simulink model "Project_Simulation"  (R2020a)
settings: Solver=ode45  StartTime=0.0  StopTime=1  RelTol=1e-3
libraries: powerlib x17, re_lib x1, simulink x1
settings Model: Creator=Kryptic  LastModifiedBy=Kryptic

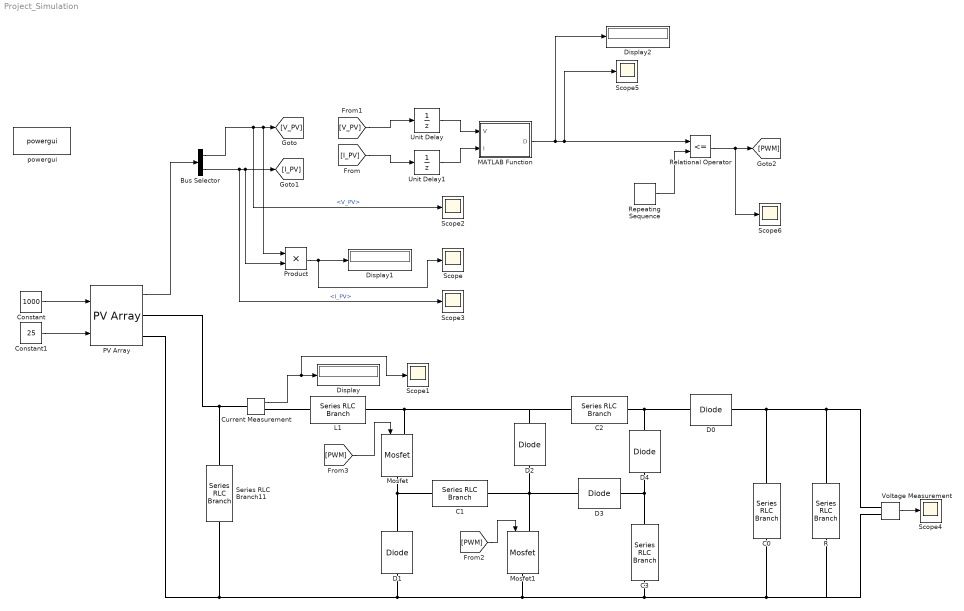
== system Project_Simulation ==
  Bus Selector : BusSelector  OutputSignals=V_PV,I_PV
  C0 : powerlib/Elements/Series RLC Branch  LConnTagsString=__new0  RConnTagsString=__new0  BranchType=C  Resistance=1  Inductance=1e-3  SetiL0=off  InitialCurrent=0  Capacitance=9.82e-8  Setx0=off  InitialVoltage=0  Measurements=None
  C1 : powerlib/Elements/Series RLC Branch  LConnTagsString=__new0  RConnTagsString=__new0  BranchType=C  Resistance=1  Inductance=1e-3  SetiL0=off  InitialCurrent=0  Capacitance=4.74e-6  Setx0=off  InitialVoltage=0  Measurements=None
  C2 : powerlib/Elements/Series RLC Branch  LConnTagsString=__new0  RConnTagsString=__new0  BranchType=C  Resistance=1  Inductance=1e-3  SetiL0=off  InitialCurrent=0  Capacitance=3.75e-7  Setx0=off  InitialVoltage=0  Measurements=None
  C3 : powerlib/Elements/Series RLC Branch  LConnTagsString=__new0  RConnTagsString=__new0  BranchType=C  Resistance=1  Inductance=1e-3  SetiL0=off  InitialCurrent=0  Capacitance=7.5e-7  Setx0=off  InitialVoltage=0  Measurements=None
  Constant : Constant  Value=1000
  Constant1 : Constant  Value=25
  Current Measurement : powerlib/Measurements/Current Measurement  PhasorSimulation=off  OutputType=Complex  PSBequivalent=0
  D0 : powerlib/Power Electronics/Diode  Ron=0.001  Lon=0  Vf=1.50  IC=0  UseSnubber=0  Rs=500  Cs=250e-9  Measurements=off
  D1 : powerlib/Power Electronics/Diode  Ron=0.001  Lon=0  Vf=0.86  IC=0  UseSnubber=0  Rs=500  Cs=250e-9  Measurements=off
  D2 : powerlib/Power Electronics/Diode  Ron=0.001  Lon=0  Vf=0.86  IC=0  UseSnubber=0  Rs=500  Cs=250e-9  Measurements=off
  D3 : powerlib/Power Electronics/Diode  Ron=0.001  Lon=0  Vf=0.86  IC=0  UseSnubber=0  Rs=500  Cs=250e-9  Measurements=off
  D4 : powerlib/Power Electronics/Diode  Ron=0.001  Lon=0  Vf=1.50  IC=0  UseSnubber=0  Rs=500  Cs=250e-9  Measurements=off
  Display : Display
  Display1 : Display
  Display2 : Display
  L1 : powerlib/Elements/Series RLC Branch  LConnTagsString=__new0  RConnTagsString=__new0  BranchType=L  Resistance=1  Inductance=20e-3  SetiL0=off  InitialCurrent=0  Capacitance=1e-6  Setx0=off  InitialVoltage=0  Measurements=None
  MATLAB Function : MATLAB Function  TreatAsAtomicUnit=on
  Mosfet : powerlib/Power Electronics/Mosfet  Ron=8e-3  Lon=0  Rd=0.01  Vfd=0  IC=0  Rs=1e5  Cs=inf  Measurements=off
  Mosfet1 : powerlib/Power Electronics/Mosfet  Ron=8e-3  Lon=0  Rd=0.01  Vfd=0  IC=0  Rs=1e5  Cs=inf  Measurements=off
  PV Array : re_lib/Solar/PV Array  Npar=1  Nser=1  PlotType=array @ 25 deg.C & specified irradiances  S_vec="[ 1000  500  100 ]"  Temp_C_vec="[ 45 25  ]"  ModuleName=User-defined  PlotWhenSelected=off  Pm=20.06  Ncell=60  Voc=21  Isc=1.2  Vm=17  Im=1.18  beta_Voc_pc=-.585  alpha_Isc_pc=0.00367  beta_Voc=-0.12285  alpha_Isc=4.404e-05  IL=1.2439  I0=1.4121e-08  nI=0.7447  Rsh=22939.389  Rs=0.77008  RobustModel=off  RobustCellTemperature=25  BAL=on  Tc=1e-6  Tfilter=5e-5
  Product : Product
  R : powerlib/Elements/Series RLC Branch  LConnTagsString=__new0  RConnTagsString=__new0  BranchType=R  Resistance=2645  Inductance=1e-3  SetiL0=off  InitialCurrent=0  Capacitance=1e-6  Setx0=off  InitialVoltage=0  Measurements=None
  Relational Operator : RelationalOperator  Operator=<=  OutDataTypeStr=boolean  RndMeth=Simplest
  Repeating Sequence : simulink/Sources/Repeating Sequence  rep_seq_t=[0 1/30000]  rep_seq_y=[0 1]
  Scope{,1..6} (7 alike) : Scope
  Series RLC Branch11 : powerlib/Elements/Series RLC Branch  LConnTagsString=__new0  RConnTagsString=__new0  BranchType=RC  Resistance=0.0001  Inductance=1e-3  SetiL0=off  InitialCurrent=0  Capacitance=1000e-6  Setx0=off  InitialVoltage=0  Measurements=None
  Unit Delay : UnitDelay  SampleTime=1e-4  HasFrameUpgradeWarning=on
  Unit Delay1 : UnitDelay  SampleTime=1e-4  HasFrameUpgradeWarning=on
  Voltage Measurement : powerlib/Measurements/Voltage Measurement  PhasorSimulation=off  OutputType=Complex  PSBequivalent=0
  powergui : powerlib/powergui  Priority=1  SimulationMode=Discrete  SampleTime=1e-6  frequency=60  Iterations=50  frequencyindice=0  Pbase=100e6  ErrMax=1e-4  UnitsV=kV  UnitsW=MW  buscounter=0  FunctionMessages=off  echomessages=off  EnableUseOfTLC=off  CurrentSourceSwitches=off  DisableSnubberDevices=off  DisableRonSwitches=off  DisableVfSwitches=off  DisplayEquations=off  AutomaticDiscreteSolvers=off  SolverType=Tustin/Backward Euler (TBE)  Interpol=off  ExternalGateDelay=off  methode=off  Ts=100  x0status=blocks  SPID=on  SwTol=0  HookPort=off  NonlinearTolerance=1e-4  nMaxIteration=100  ContinueOnMaxIteration=off  RestoreLinks=warning  ResistiveCurrentMeasurement=off  Frange=[0:2:500]  Ylog=off  Xlog=on  ShowGrid=off  save=off  variable=ZData  structure=0  ZoomFFT=off  StartTime=0.0  cycles=1  DisplayStyle=1  fundamental=60  FreqAxis=off  MaxFrequency=1000  frequencyindicesteady=1  RmsSteady=1  display=off
  wires:
  Constant1/1 -> PV Array/2
  Constant/1 -> PV Array/1
  PV Array/1 -> Bus Selector/1
  Bus Selector/2 -> Scope3/1, [I_PV], Product/2  "<I_PV>"
  Bus Selector/1 -> [V_PV], Product/1, Scope2/1  "<V_PV>"
  [V_PV] -> Unit Delay/1
  [I_PV] -> Unit Delay1/1
  Repeating Sequence/1 -> Relational Operator/2
  Relational Operator/1 -> Scope6/1, [PWM]
  [PWM] -> Mosfet/1
  [PWM] -> Mosfet1/1
  Unit Delay/1 -> MATLAB Function/1(V)
  Unit Delay1/1 -> MATLAB Function/2(I)
  MATLAB Function/1(D) -> Display2/1, Scope5/1, Relational Operator/1
  Current Measurement/1 -> Scope1/1, Display/1
  Product/1 -> Scope/1, Display1/1
  Voltage Measurement/1 -> Scope4/1
  connections:
  PV Array/RConn1 -- Current Measurement/LConn1 -- Series RLC Branch11/LConn1
  PV Array/RConn2 -- D1/RConn1 -- C0/RConn1 -- R/RConn1 -- Voltage Measurement/LConn2 -- C3/RConn1 -- Mosfet1/RConn1 -- Series RLC Branch11/RConn1
  Mosfet/LConn1 -- C2/LConn1 -- D2/LConn1 -- L1/RConn1
  D1/LConn1 -- C1/LConn1 -- Mosfet/RConn1
  Mosfet1/LConn1 -- C1/RConn1 -- D2/RConn1 -- D3/LConn1
  D0/LConn1 -- C2/RConn1 -- D4/RConn1
  D3/RConn1 -- D4/LConn1 -- C3/LConn1
  R/LConn1 -- Voltage Measurement/LConn1 -- D0/RConn1 -- C0/LConn1
  Current Measurement/RConn1 -- L1/LConn1

== matlab function Project_Simulation/MATLAB Function ==
  data: V input; D output; I input
function D = DutyRatio(V, I)

Dmax = 0.95;
Dmin = 0;
Dinit = 0.95;
deltaD = 0.001;
persistent  Vold Pold Dold;

dataType = 'double';

if isempty(Vold)
    Vold = 0;
    Pold = 0;
    Dold = Dinit;
end

P = V*I;
dV = V-Vold;
dP = P-Pold;

if dP ~= 0
    if dP<0
        if dV<0
            D = Dold + deltaD;
        else
            D = Dold - deltaD;
        end
    else
        if dV<0
            D =Dold + deltaD;
        else
            D = Dold - deltaD;
        end
    end
else D = Dold;
end

if D >= Dmax | D <= Dmin
    D=Dold;
end

Dold = D;
Vold = V;
Pold = P;
